simulink model "discreteSystem"  (R2020b)
settings: Solver=VariableStepAuto  StartTime=0.0  StopTime=10.0  RelTol=1e-3
values from neighbouring files (symbols this model uses):
  K_phi = 2.93    [stepResponse.m]
  K_rho = 40.8    [stepResponse.m]
  sigma_phi = 6.061    [stepResponse.m]
  sigma_rho = 5.305    [stepResponse.m]
undefined symbols (not defined in the file or in its folder): rho_dot_set, x_s, y_s
settings Model: Creator=mini-  LastModifiedBy=mini-

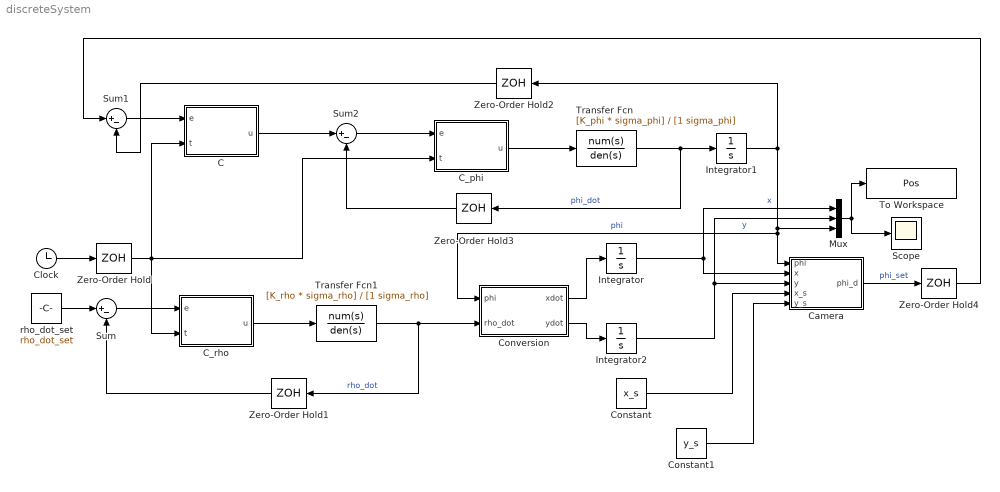
== system discreteSystem ==
  C : MATLAB Function  TreatAsAtomicUnit=on
  C_phi : MATLAB Function  TreatAsAtomicUnit=on
  C_rho : MATLAB Function  TreatAsAtomicUnit=on
  Camera : MATLAB Function  TreatAsAtomicUnit=on
  Clock : Clock
  Constant : Constant  Value=x_s
  Constant1 : Constant  Value=y_s
  Conversion : MATLAB Function  TreatAsAtomicUnit=on
  Integrator : Integrator
  Integrator1 : Integrator
  Integrator2 : Integrator
  Mux : Mux  Inputs=3
  Scope : Scope
  Sum : Sum  Inputs=|+-
  Sum1 : Sum  Inputs=|+-
  Sum2 : Sum  Inputs=|+-
  To Workspace : ToWorkspace  VariableName=Pos  SaveFormat=Timeseries  SampleTime=-1
  Transfer Fcn : TransferFcn  Numerator=[K_phi * sigma_phi]  Denominator=[1 sigma_phi]
  Transfer Fcn1 : TransferFcn  Numerator=[K_rho * sigma_rho]  Denominator=[1 sigma_rho]
  Zero-Order Hold{,1..4} (5 alike) : ZeroOrderHold  SampleTime=-1
  rho_dot_set : Constant  Value=rho_dot_set
  wires:
  rho_dot_set/1 -> Sum/1
  Sum/1 -> C_rho/1(e)
  C_rho/1(u) -> Transfer Fcn1/1
  Transfer Fcn1/1 -> Conversion/2(rho_dot), Zero-Order Hold1/1  "rho_dot"
  Zero-Order Hold1/1 -> Sum/2
  Clock/1 -> Zero-Order Hold/1
  Sum1/1 -> C/1(e)
  Zero-Order Hold2/1 -> Sum1/2
  C_phi/1(u) -> Transfer Fcn/1
  C/1(u) -> Sum2/1
  Transfer Fcn/1 -> Integrator1/1, Zero-Order Hold3/1  "phi_dot"
  Zero-Order Hold3/1 -> Sum2/2
  Sum2/1 -> C_phi/1(e)
  Integrator1/1 -> Zero-Order Hold2/1, Camera/1(phi), Conversion/1(phi), Mux/3  "phi"
  Camera/1(phi_d) -> Zero-Order Hold4/1  "phi_set"
  Zero-Order Hold4/1 -> Sum1/1
  Conversion/1(xdot) -> Integrator/1
  Conversion/2(ydot) -> Integrator2/1
  Zero-Order Hold/1 -> C/2(t), C_phi/2(t), C_rho/2(t)
  Integrator/1 -> Mux/1, Camera/2(x)  "x"
  Integrator2/1 -> Mux/2, Camera/3(y)  "y"
  Constant/1 -> Camera/4(x_s)
  Constant1/1 -> Camera/5(y_s)
  Mux/1 -> Scope/1, To Workspace/1

== matlab function discreteSystem/C_rho ==
  data: e input; u output; t input
function u = fcn(e,t)
%% Define Variables
% Control Gains
Kp=1;
Ki=5;
umax = 10;
% Memory variables
persistent I_past;
persistent t_past;
if isempty(I_past), I_past=0; end;
if isempty(t_past), t_past=0; end;
%% Calculate Controller output
% sample time
Ts = t - t_past;
% Integrator
I = I_past+e*Ts;
% PI control calculation
u = Kp*e+Ki*I;
% anti-windup6
if abs(u)>umax,
    u = sign(u)*umax;
    e = sign(e)*min(umax/Kp, abs(e));
    I = (u-Kp*e)/Ki;
end;
I_past=I;
t_past=t;

== matlab function discreteSystem/C ==
  data: e input; u output; t input
function u = fcn(e,t)
%% Define Variables
% Control Gains
Kp = 10;
Kd = 0.25;
% Memory variables
persistent t_past;
persistent e_past;
if isempty(t_past), t_past=0; end;
if isempty(e_past), e_past=0; end;
%% Calculate Controller output
% sample time
Ts = t - t_past;
% Differentiator
if Ts > 0
    D = (e - e_past)/Ts;
else
    D = 0;
end
% PI control calculation
u = Kp*e+Kd*D;
t_past=t;
e_past=e;

== matlab function discreteSystem/C_phi ==
  data: e input; u output; t input
function u = fcn(e,t)
%% Define Variables
% Control Gains
Kp=0.1;
Ki=1;
umax = 10;
% Memory variables
persistent I_past;
persistent t_past;
if isempty(I_past), I_past=0; end;
if isempty(t_past), t_past=0; end;
%% Calculate Controller output
% sample time
Ts = t - t_past;
% Integrator
I = I_past+e*Ts;
% PI control calculation
u = Kp*e+Ki*I;
% anti-windup6
if abs(u)>umax,
    u = sign(u)*umax;
    e = sign(e)*min(umax/Kp, abs(e));
    I = (u-Kp*e)/Ki;
end;
I_past=I;
t_past=t;

== matlab function discreteSystem/Conversion ==
  data: phi input; xdot output; rho_dot input; ydot output
function [xdot,ydot] = fcn(phi,rho_dot)
xdot = rho_dot * cos(phi);
ydot = rho_dot * sin(phi);

== matlab function discreteSystem/Camera ==
  data: phi input; phi_d output; x input; y input; x_s input; y_s input
function phi_d = fcn(phi,x,y,x_s,y_s)
phi_s = atan2(y_s-y,x_s-x) - phi;
phi_d = phi + phi_s;
